simulink library "animation_lib"  (Simulink 7.8)
settings: Solver=ode45  SolverMode=SingleTasking  StartTime=0.0  StopTime=10.0  RelTol=1e-3
PostLoadFcn:
  | load_system('aerolibv1')
  | setsysloc('aerolibv1')
Description:
  | Aerospace Blockset Library: MATLAB-Based Animation
settings Model: FPTRunName=Active  Creator=The MathWorks Inc.  LastModifiedBy=sven  ExtModeAutoUpdateStatusClock=off

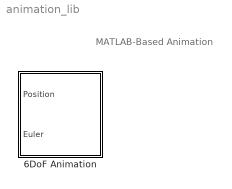
== system animation_lib ==
  note: MATLAB-Based Animation
  6DoF Animation : Subsystem  TreatAsAtomicUnit=on  SimViewingDevice=on  mask(6DoF_Animation){u1=[0 4000 -2000 2000 -5000 -3000], u2=0.1, u3=1.0, u4=[4000 0 -5000], u5=Fixed position, u6=[2000 500 -3150], u7=10, u8=on}
      mask prompts: u1 "Axes limits [xmin xmax ymin ymax zmin zmax]:"; u2 "Time interval between updates:"; u3 "Size of craft displayed:"; u4 "Static object position [xp yp zp]:"; u5 "Enter view:"; u6 "Position of camera [xc yc zc]:"; u7 "View angle:"; u8 "Enable animation"
      mask help:
      | Create a 3-D animated view of a six-degrees-of-freedom craft, where X, Y, and Z craft position (Position) and craft Euler angles (Euler) are inputs.
      |
      | Display parameters are in the same units of length as the input parameters.
      mask init:
      | Config.axes = u1;
      | Config.update = u2;
      | Config.craft = u3;
      | Config.target = u4;
      | Config.camera_view = u5;
      | Config.camera_pos = u6;
      | Config.view = u7;
      | Config.Animenable = u8;
      | [xp yp] = aeroimage('anim',gcbh);
      mask Help: eval('asbhelp(''sixdof_animation'')');
      mask StyleString: edit,edit,edit,edit,popup(Fixed position|Cockpit|Fly alongside),edit,edit,checkbox
      mask Display:
      | port_label('input',1,'x_e','texmode','on');
      | port_label('input',2,'\phi \theta \psi','texmode','on');
      | patch(xp,yp)

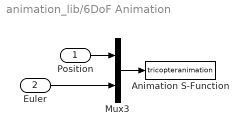
== system animation_lib/6DoF Animation ==
  Position : Inport
  Euler : Inport  Port=2
  Animation S-Function : S-Function  FunctionName=tricopteranimation  Parameters=Config  EnableBusSupport=off
  Mux3 : Mux  Inputs=2
  wires:
  Euler/1 -> Mux3/2
  Position/1 -> Mux3/1
  Mux3/1 -> Animation S-Function/1
